simulink model "project_simulink"  (R2024a)
settings: Solver=VariableStepAuto  StartTime=0.0  StopTime=100  RelTol=1e-3
values from neighbouring files (symbols this model uses):
  b = 9.144    [aircraft_6dof.m]
  c = 3.45    [aircraft_6dof.m]
  delta_lef = 0    [aircraft_6dof.m]
  delta_r = 0    [aircraft_6dof.m]
  delta_sb = 0    [aircraft_6dof.m]
  f16_database =     [F16_LookupTables.mat]
  mass = 9300    [aircraft_6dof.m]
  S = 27.88    [aircraft_6dof.m]
  V_c = [153]    [aircraft_6dof.m]
libraries: aerolibconvert2 x5, shared6dof x1, aerolibatmos2 x1, aerolibasang x1
(part 1 of 2)
settings Model: Creator=caner  LastModifiedBy=HUSEYIN
settings OptimizationCC: ReuseModelBlockBuffer=off
settings RTWCC: GPUComputeCapability=3.5

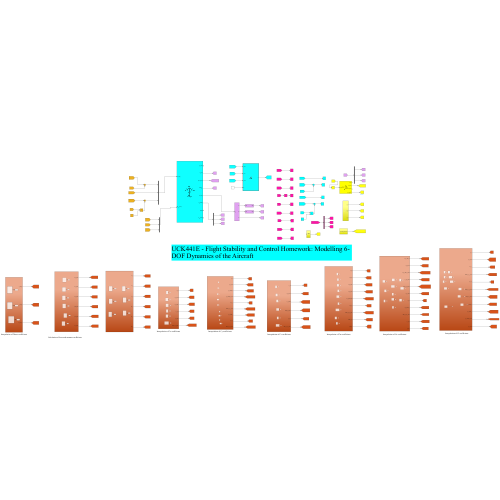
[thumbnail: Simulink's stored preview of the top-level diagram]
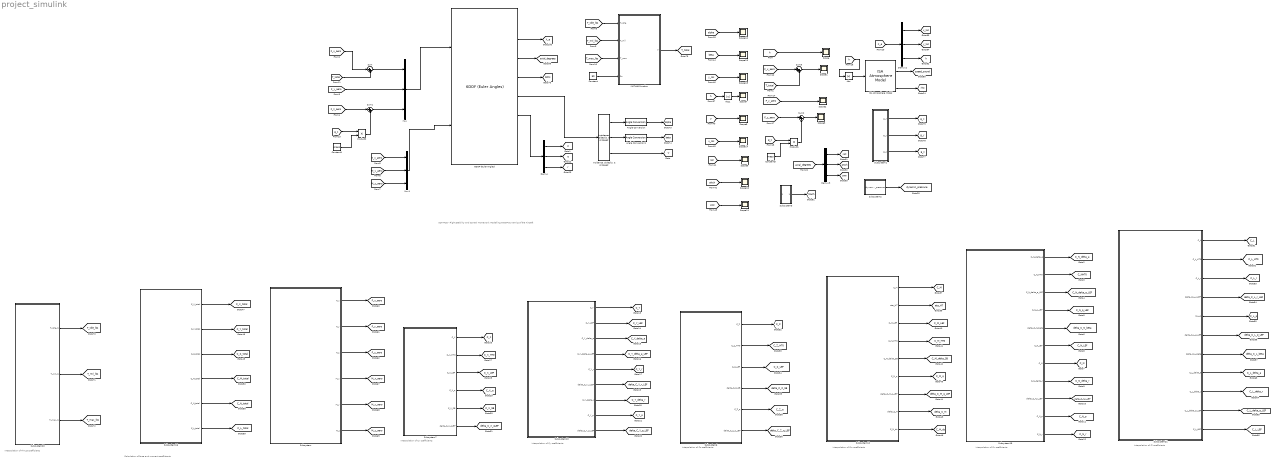
== system project_simulink ==
  note: UCK441E - Flight Stability and Control Homework: Modelling 6-DOF Dynamics of the Aircraft
  note: Interpolation of Cx coefficients
  note: Interpolation of Cy coefficients
  note: Interpolation of Cz coefficients
  note: Interpolation of Cm coefficients
  note: Interpolation of Cn coefficients
  note: Interpolation of Cl coefficients
  note: Interpolation of Thrust coefficients
  note: Calculation of force and moment coefficients
  6DOF (Euler Angles) : shared6dof/6DOF (Euler Angles)  units=Metric (MKS)  mtype=Fixed  rep=Euler Angles  xme_0=[0 0 -3048]  Vm_0=[153 0 0]  eul_0=[0 0 0]  pm_0=[0 0 0]  mass_0=9300  mass_e=0.5  mass_f=2.0  inertia=I  inertia_e=eye(3)  inertia_f=2*eye(3)  k_quat=1.0  vre_flag=on  abi_flag=off  aMode=0  xme_statename=''  Vm_statename=''  eul_statename=''  quat_statename=''  pm_statename=''  mass_statename=''
  Abs : Abs  SaturateOnIntegerOverflow=off
  Abs1 : Abs  SaturateOnIntegerOverflow=off
  Angle Conversion : aerolibconvert2/Angle Conversion  IU=rad  OU=deg
  Angle Conversion1 : aerolibconvert2/Angle Conversion  IU=rad  OU=deg
  Constant : Constant  Value=50
  Constant1 : Constant  Value=mass
  Constant3 : Constant  Value=mass
  Demux : Demux  Outputs=3
  Demux2 : Demux  Outputs=3
  Demux3 : Demux  Outputs=3
  ISA Atmosphere Model : aerolibatmos2/ISA Atmosphere Model  useExtended=off  action=Warning  custom=off  viscosityOut=off  g=9.80665  gamma=1.4  R=287.0531  L=0.0065  h_trop=11000  h_strat=20000  rho0=1.225  P0=101325  T0=288.15  h0=0  S=110.4  Tref=273.15  muref=1.716e-5
  "Incidence, Sideslip, & Airspeed" : aerolibasang/Incidence, Sideslip, & Airspeed
  MATLAB Function : MATLAB Function  TreatAsAtomicUnit=on
  Mux : Mux  Inputs=3
  Mux1 : Mux  Inputs=3
  Product1 : Product
  Product2 : Product
  Scope{,1..3,7..15} (13 alike) : Scope
  Subsystem : Subsystem
  Subsystem1 : Subsystem
  Subsystem10 : Subsystem
  Subsystem12 : Subsystem
  Subsystem15 : Subsystem
  Subsystem16 : Subsystem
  Subsystem2 : Subsystem
  Subsystem20 : Subsystem
  Subsystem21 : Subsystem
  Subsystem3 : Subsystem
  Subsystem6 : Subsystem
  Subsystem7 : Subsystem
  Sum{,1..3} (4 alike) : Sum  Inputs=|++
  tag scope: C_L=global, C_L_HT0=global, C_L_LEF=global, C_L_delta_a=global, C_L_delta_a_LEF=global, C_L_delta_r=global, C_L_p=global, C_L_r=global, C_L_total=global, C_M=global, C_M_HT0=global, C_M_LEF=global, C_M_delta_SB=global, C_M_ds=global, C_M_q=global, C_M_total=global, C_N=global, C_NHT0=global, C_N_LEF=global, C_N_delta_a=global, C_N_delta_a_LEF=global, C_N_delta_r=global, C_N_p=global, C_N_p_LEF=global, C_N_r=global, C_N_total=global, C_X=global, C_X_HT0=global, C_X_LEF=global, C_X_SB=global, C_X_q=global, C_X_total=global, C_Y=global, C_Y_LEF=global, C_Y_delta_a=global, C_Y_delta_a_LEF=global, C_Y_delta_r=global, C_Y_p=global, C_Y_r=global, C_Y_total=global, C_Z=global, C_Z_HT0=global, C_Z_LEF=global, C_Z_q=global, C_Z_total=global, DCM=global, F_x_aero=global, F_y_aero=global, F_z_aero=global, M_x_aero=global, M_y_aero=global, M_z_aero=global, Mach=global, T_idle_lbs=global, T_max_lbs=global, T_mil_lbs=global, T_total=global, V=global, X_e=global, alpha=global, axial_degrees=global, beta=global, delta_C_L_beta=global, delta_C_L_p_LEF=global, delta_C_L_r_LEF=global, delta_C_M=global, delta_C_M_q_LEF=global, delta_C_N_beta=global, delta_C_N_r_LEF=global, delta_C_X_qLEF=global, delta_C_Y_p_LEF=global, delta_C_Y_r_LEF=global, delta_C_Z_SB=global, delta_C_Z_q_LEF=global, dynamic_pressure=global, eta_HT=global, g_x=global, g_y=global, g_z=global, h=global, p=global, pitch=global, q=global, r=global, rho=global, roll=global, speed_sound=global, x_loc=global, y_loc=global, yaw=global
  wires:
  6DOF (Euler Angles)/5 -> "Incidence, Sideslip, & Airspeed"/1
  "Incidence, Sideslip, & Airspeed"/3 -> [V]
  6DOF (Euler Angles)/6 -> Demux/1
  Subsystem15/1(C_N_delta_a) -> [C_N_delta_a]
  Subsystem15/3(C_N_delta_a_LEF) -> [C_N_delta_a_LEF]
  Subsystem15/4(C_N_p_LEF) -> [C_N_p_LEF]
  Subsystem15/5(delta_C_N_beta) -> [delta_C_N_beta]
  Subsystem15/7(C_N) -> [C_N]
  Subsystem15/6(C_N_LEF) -> [C_N_LEF]
  Subsystem15/2(C_N_HT0) -> [C_NHT0]
  Subsystem15/8(C_N_delta_r) -> [C_N_delta_r]
  Subsystem15/9(delta_C_N_r_LEF) -> [delta_C_N_r_LEF]
  Subsystem15/10(C_N_p) -> [C_N_p]
  Subsystem15/11(C_N_r) -> [C_N_r]
  Subsystem10/1(C_Y) -> [C_Y]
  Subsystem10/2(C_Y_LEF) -> [C_Y_LEF]
  Subsystem10/3(C_Y_delta_a) -> [C_Y_delta_a]
  Subsystem10/4(C_Y_delta_a_LEF) -> [C_Y_delta_a_LEF]
  Subsystem10/5(C_Y_r) -> [C_Y_r]
  Subsystem10/6(delta_C_Y_r_LEF) -> [delta_C_Y_r_LEF]
  Subsystem10/7(C_Y_delta_r) -> [C_Y_delta_r]
  Subsystem10/8(C_Y_p) -> [C_Y_p]
  Subsystem10/9(delta_C_Y_p_LEF) -> [delta_C_Y_p_LEF]
  ISA Atmosphere Model/4 -> [rho]
  Subsystem7/1(C_X) -> [C_X]
  Subsystem7/2(C_X_HT0) -> [C_X_HT0]
  Subsystem7/3(C_X_LEF) -> [C_X_LEF]
  Subsystem7/4(C_X_q) -> [C_X_q]
  Subsystem7/5(C_X_SB) -> [C_X_SB]
  Subsystem7/6(delta_C_X_qLEF) -> [delta_C_X_qLEF]
  Subsystem6/1(C_Z) -> [C_Z]
  Subsystem6/2(C_Z_HT0) -> [C_Z_HT0]
  Subsystem6/3(C_Z_LEF) -> [C_Z_LEF]
  Subsystem6/4(delta_C_Z_SB) -> [delta_C_Z_SB]
  Subsystem6/5(C_Z_q) -> [C_Z_q]
  Subsystem6/6(delta_C_Z_q_LEF) -> [delta_C_Z_q_LEF]
  Subsystem12/1(C_M) -> [C_M]
  Subsystem12/2(eta_HT) -> [eta_HT]
  Subsystem12/3(C_M_LEF) -> [C_M_LEF]
  Subsystem12/4(C_M_HT0) -> [C_M_HT0]
  Subsystem12/5(C_M_delta_SB) -> [C_M_delta_SB]
  Subsystem12/6(C_M_q) -> [C_M_q]
  Subsystem12/7(delta_C_M_q_LEF) -> [delta_C_M_q_LEF]
  Subsystem12/8(delta_C_M) -> [delta_C_M]
  Subsystem12/9(C_M_ds) -> [C_M_ds]
  Subsystem21/1(C_L) -> [C_L]
  Subsystem21/2(C_L_HT0) -> [C_L_HT0]
  Subsystem21/3(C_L_r) -> [C_L_r]
  Subsystem21/4(delta_C_L_r_LEF) -> [delta_C_L_r_LEF]
  Subsystem21/5(C_L_p) -> [C_L_p]
  Subsystem21/6(delta_C_L_p_LEF) -> [delta_C_L_p_LEF]
  Subsystem21/7(delta_C_L_beta) -> [delta_C_L_beta]
  Subsystem21/8(C_L_delta_a) -> [C_L_delta_a]
  Subsystem21/9(C_L_delta_r) -> [C_L_delta_r]
  Subsystem21/10(C_L_delta_a_LEF) -> [C_L_delta_a_LEF]
  Subsystem21/11(C_L_LEF) -> [C_L_LEF]
  [F_y_aero] -> Mux/2
  Mux/1 -> 6DOF (Euler Angles)/1
  [M_x_aero] -> Mux1/1
  [M_z_aero] -> Mux1/3
  [M_y_aero] -> Mux1/2
  Mux1/1 -> 6DOF (Euler Angles)/2
  Subsystem20/1(T_idle_N) -> [T_idle_lbs]
  Subsystem20/2(T_mil_N) -> [T_mil_lbs]
  Subsystem20/3(T_max_N) -> [T_max_lbs]
  Subsystem16/1(C_X_total) -> [C_X_total]
  Subsystem16/2(C_Y_total) -> [C_Y_total]
  Subsystem16/3(C_Z_total) -> [C_Z_total]
  Subsystem16/4(C_M_total) -> [C_M_total]
  Subsystem16/5(C_N_total) -> [C_N_total]
  Subsystem16/6(C_L_total) -> [C_L_total]
  Subsystem/1(F_x) -> [F_x_aero]
  Subsystem/2(F_y) -> [F_y_aero]
  Subsystem/3(F_z) -> [F_z_aero]
  Subsystem/4(M_x) -> [M_x_aero]
  Subsystem/5(M_y) -> [M_y_aero]
  Subsystem/6(M_z) -> [M_z_aero]
  "Incidence, Sideslip, & Airspeed"/1 -> Angle Conversion/1
  Angle Conversion/1 -> [alpha]
  "Incidence, Sideslip, & Airspeed"/2 -> Angle Conversion1/1
  Angle Conversion1/1 -> [beta]
  Demux/1 -> [p]
  Demux/2 -> [q]
  Demux/3 -> [r]
  [T_idle_lbs] -> MATLAB Function/1(T_idle)
  [T_mil_lbs] -> MATLAB Function/2(T_mil)
  [T_max_lbs] -> MATLAB Function/3(T_max)
  Constant/1 -> MATLAB Function/4(Pc)
  MATLAB Function/1(T) -> [T_total]
  [F_x_aero] -> Sum/1
  [T_total] -> Sum/2
  Sum/1 -> Mux/1
  6DOF (Euler Angles)/4 -> [DCM]
  [F_z_aero] -> Sum1/1
  [g_z] -> Product2/1
  Constant1/1 -> Product2/2
  Sum1/1 -> Mux/3
  Product2/1 -> Sum1/2
  ISA Atmosphere Model/2 -> [speed_sound]
  Demux2/3 -> [h]
  Demux2/1 -> [x_loc]
  Demux2/2 -> [y_loc]
  Subsystem1/1(g_x) -> [g_x]
  Subsystem1/2(g_y) -> [g_y]
  Subsystem1/3(g_z) -> [g_z]
  Subsystem2/1(dynamic_pressure) -> [dynamic_pressure]
  Subsystem3/1(Mach) -> [Mach]
  [T_total] -> Sum3/2
  [F_x_aero] -> Sum3/1
  Product1/1 -> Sum2/2
  Sum2/1 -> Scope3/1
  Constant3/1 -> Product1/2
  [F_z_aero] -> Sum2/1
  [g_z] -> Product1/1
  Sum3/1 -> Scope1/1
  [F_y_aero] -> Scope2/1
  [h] -> Abs/1
  Abs/1 -> ISA Atmosphere Model/1
  [h] -> Scope/1
  6DOF (Euler Angles)/2 -> [X_e]
  [X_e] -> Demux2/1
  6DOF (Euler Angles)/3 -> [axial_degrees]
  [axial_degrees] -> Demux3/1
  Demux3/1 -> [roll]
  Demux3/2 -> [pitch]
  Demux3/3 -> [yaw]
  [V] -> Scope8/1
  Abs1/1 -> Scope7/1
  [h] -> Abs1/1
  [roll] -> Scope9/1
  [pitch] -> Scope10/1
  [yaw] -> Scope11/1
  [alpha] -> Scope12/1
  [beta] -> Scope13/1
  [x_loc] -> Scope14/1
  [y_loc] -> Scope15/1

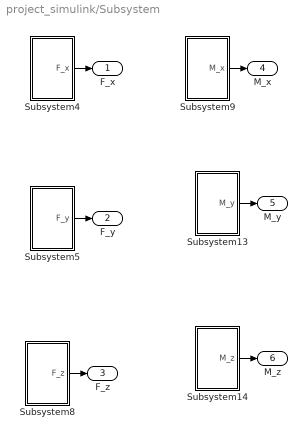
== system project_simulink/Subsystem ==
  Subsystem13 : Subsystem
  Subsystem14 : Subsystem
  Subsystem4 : Subsystem
  Subsystem5 : Subsystem
  Subsystem8 : Subsystem
  Subsystem9 : Subsystem
  F_x : Outport
  F_y : Outport  Port=2
  F_z : Outport  Port=3
  M_x : Outport  Port=4
  M_y : Outport  Port=5
  M_z : Outport  Port=6
  wires:
  Subsystem14/1(M_z) -> M_z/1
  Subsystem4/1(F_x) -> F_x/1
  Subsystem8/1(F_z) -> F_z/1
  Subsystem13/1(M_y) -> M_y/1
  Subsystem5/1(F_y) -> F_y/1
  Subsystem9/1(M_x) -> M_x/1

== system project_simulink/Subsystem1 ==
  Demux1 : Demux  Outputs=3
  Product1 : Product  Multiplication=Matrix(*)
  gravitational acceleration : Constant  Value=[0,0,9.81]
  g_x : Outport
  g_y : Outport  Port=2
  g_z : Outport  Port=3
  wires:
  gravitational acceleration/1 -> Product1/2
  Demux1/2 -> g_y/1  "g_y"
  Product1/1 -> Demux1/1
  Demux1/3 -> g_z/1  "g_z"
  [DCM] -> Product1/1
  Demux1/1 -> g_x/1  "g_x"

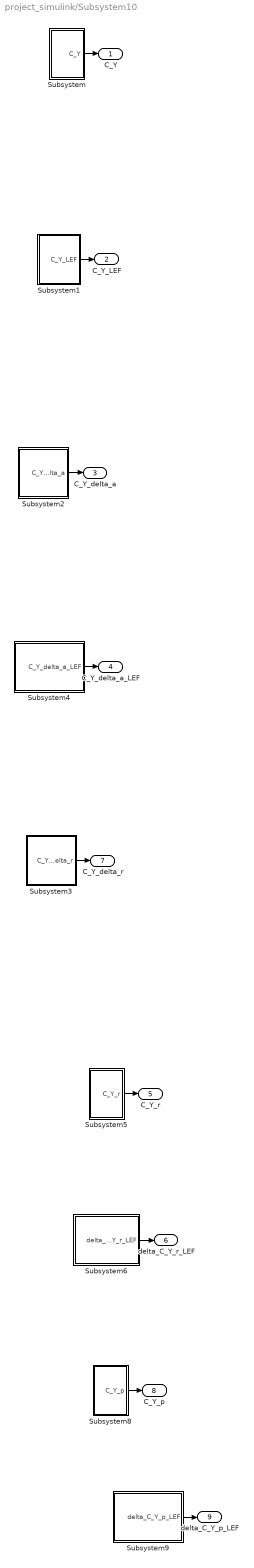
== system project_simulink/Subsystem10 ==
  Subsystem : Subsystem
  Subsystem1 : Subsystem
  Subsystem2 : Subsystem
  Subsystem3 : Subsystem
  Subsystem4 : Subsystem
  Subsystem5 : Subsystem
  Subsystem6 : Subsystem
  Subsystem8 : Subsystem
  Subsystem9 : Subsystem
  C_Y : Outport
  C_Y_LEF : Outport  Port=2
  C_Y_delta_a : Outport  Port=3
  C_Y_delta_a_LEF : Outport  Port=4
  C_Y_r : Outport  Port=5
  delta_C_Y_r_LEF : Outport  Port=6
  C_Y_delta_r : Outport  Port=7
  C_Y_p : Outport  Port=8
  delta_C_Y_p_LEF : Outport  Port=9
  wires:
  Subsystem2/1(C_Y_delta_a) -> C_Y_delta_a/1
  Subsystem/1(C_Y) -> C_Y/1
  Subsystem1/1(C_Y_LEF) -> C_Y_LEF/1
  Subsystem6/1(delta_C_Y_r_LEF) -> delta_C_Y_r_LEF/1
  Subsystem4/1(C_Y_delta_a_LEF) -> C_Y_delta_a_LEF/1
  Subsystem9/1(delta_C_Y_p_LEF) -> delta_C_Y_p_LEF/1
  Subsystem5/1(C_Y_r) -> C_Y_r/1
  Subsystem3/1(C_Y_delta_r) -> C_Y_delta_r/1
  Subsystem8/1(C_Y_p) -> C_Y_p/1

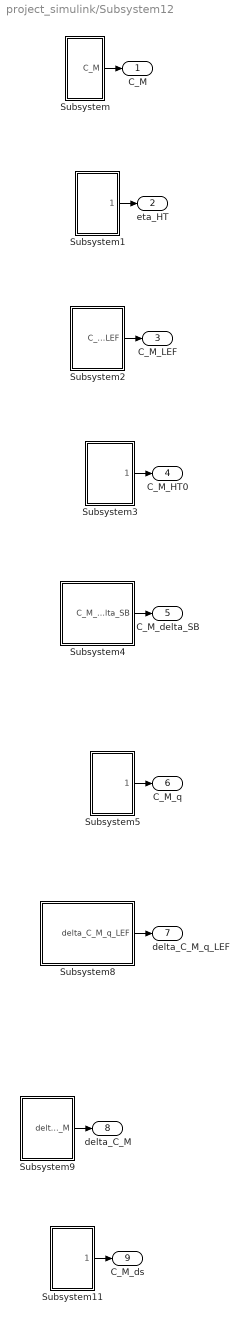
== system project_simulink/Subsystem12 ==
  Subsystem : Subsystem
  Subsystem1 : Subsystem
  Subsystem11 : Subsystem
  Subsystem2 : Subsystem
  Subsystem3 : Subsystem
  Subsystem4 : Subsystem
  Subsystem5 : Subsystem
  Subsystem8 : Subsystem
  Subsystem9 : Subsystem
  C_M : Outport
  eta_HT : Outport  Port=2
  C_M_LEF : Outport  Port=3
  C_M_HT0 : Outport  Port=4
  C_M_delta_SB : Outport  Port=5
  C_M_q : Outport  Port=6
  delta_C_M_q_LEF : Outport  Port=7
  delta_C_M : Outport  Port=8
  C_M_ds : Outport  Port=9
  wires:
  Subsystem4/1(C_M_delta_SB) -> C_M_delta_SB/1
  Subsystem5/1(C_M_q) -> C_M_q/1
  Subsystem8/1(delta_C_M_q_LEF) -> delta_C_M_q_LEF/1
  Subsystem1/1(eta_HT) -> eta_HT/1
  Subsystem11/1(C_M_ds) -> C_M_ds/1
  Subsystem/1(C_M) -> C_M/1
  Subsystem3/1(C_M_HT0) -> C_M_HT0/1
  Subsystem2/1(C_M_LEF) -> C_M_LEF/1
  Subsystem9/1(delta_C_M) -> delta_C_M/1

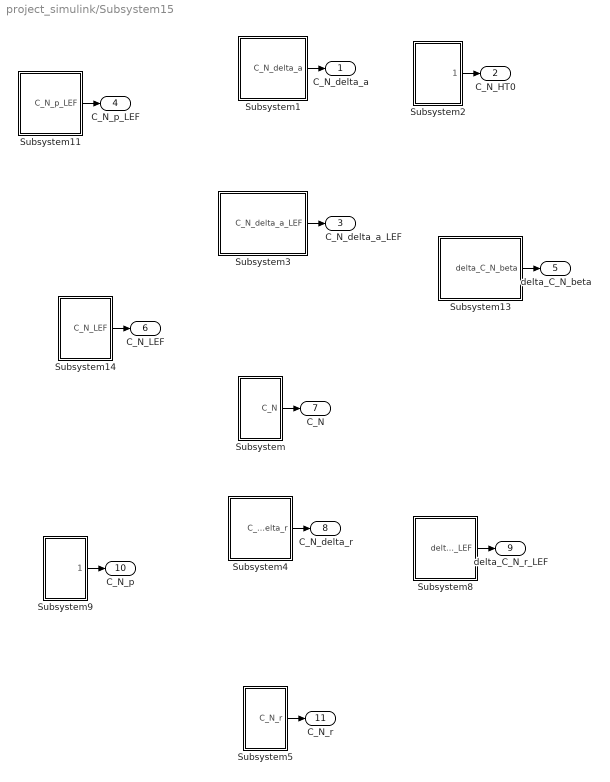
== system project_simulink/Subsystem15 ==
  Subsystem : Subsystem
  Subsystem1 : Subsystem
  Subsystem11 : Subsystem
  Subsystem13 : Subsystem
  Subsystem14 : Subsystem
  Subsystem2 : Subsystem
  Subsystem3 : Subsystem
  Subsystem4 : Subsystem
  Subsystem5 : Subsystem
  Subsystem8 : Subsystem
  Subsystem9 : Subsystem
  C_N_delta_a : Outport
  C_N_HT0 : Outport  Port=2
  C_N_delta_a_LEF : Outport  Port=3
  C_N_p_LEF : Outport  Port=4
  delta_C_N_beta : Outport  Port=5
  C_N_LEF : Outport  Port=6
  C_N : Outport  Port=7
  C_N_delta_r : Outport  Port=8
  delta_C_N_r_LEF : Outport  Port=9
  C_N_p : Outport  Port=10
  C_N_r : Outport  Port=11
  wires:
  Subsystem2/1(C_N_HT0) -> C_N_HT0/1
  Subsystem5/1(C_N_r) -> C_N_r/1
  Subsystem14/1(C_N_LEF) -> C_N_LEF/1
  Subsystem4/1(C_N_delta_r) -> C_N_delta_r/1
  Subsystem/1(C_N) -> C_N/1
  Subsystem3/1(C_N_delta_a_LEF) -> C_N_delta_a_LEF/1
  Subsystem11/1(C_N_p_LEF) -> C_N_p_LEF/1
  Subsystem9/1(C_N_p) -> C_N_p/1
  Subsystem13/1(delta_C_N_beta) -> delta_C_N_beta/1
  Subsystem1/1(C_N_delta_a) -> C_N_delta_a/1
  Subsystem8/1(delta_C_N_r_LEF) -> delta_C_N_r_LEF/1

== system project_simulink/Subsystem16 ==
  Subsystem : Subsystem
  Subsystem1 : Subsystem
  Subsystem11 : Subsystem
  Subsystem18 : Subsystem
  Subsystem2 : Subsystem
  Subsystem3 : Subsystem
  C_X_total : Outport
  C_Y_total : Outport  Port=2
  C_Z_total : Outport  Port=3
  C_M_total : Outport  Port=4
  C_N_total : Outport  Port=5
  C_L_total : Outport  Port=6
  wires:
  Subsystem18/1(C_L_total) -> C_L_total/1
  Subsystem/1(C_Y_total) -> C_Y_total/1
  Subsystem1/1(C_X_total) -> C_X_total/1
  Subsystem11/1(C_N_total) -> C_N_total/1
  Subsystem3/1(C_M_total) -> C_M_total/1
  Subsystem2/1(C_Z_total) -> C_Z_total/1

== system project_simulink/Subsystem2 ==
  Multiply : Gain  Gain=1/2
  Product : Product
  Square : Math  Operator=square
  dynamic_pressure : Outport
  wires:
  [rho] -> Product/2
  Multiply/1 -> Product/1
  Square/1 -> Multiply/1
  Product/1 -> dynamic_pressure/1  "dynamic_pressure"
  [V] -> Square/1

== system project_simulink/Subsystem20 ==
  Subsystem16 : Subsystem
  Subsystem17 : Subsystem
  Subsystem19 : Subsystem
  T_idle_N : Outport
  T_mil_N : Outport  Port=2
  T_max_N : Outport  Port=3
  wires:
  Subsystem17/1(T_mil_N) -> T_mil_N/1
  Subsystem19/1(T_max_N) -> T_max_N/1
  Subsystem16/1(T_idle_N) -> T_idle_N/1

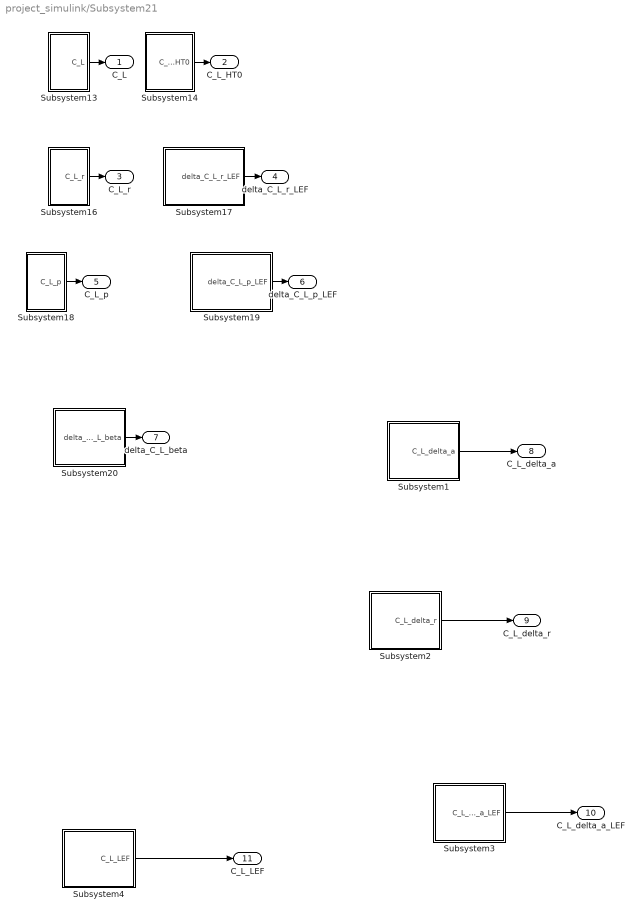
== system project_simulink/Subsystem21 ==
  Subsystem1 : Subsystem
  Subsystem13 : Subsystem
  Subsystem14 : Subsystem
  Subsystem16 : Subsystem
  Subsystem17 : Subsystem
  Subsystem18 : Subsystem
  Subsystem19 : Subsystem
  Subsystem2 : Subsystem
  Subsystem20 : Subsystem
  Subsystem3 : Subsystem
  Subsystem4 : Subsystem
  C_L : Outport
  C_L_HT0 : Outport  Port=2
  C_L_r : Outport  Port=3
  delta_C_L_r_LEF : Outport  Port=4
  C_L_p : Outport  Port=5
  delta_C_L_p_LEF : Outport  Port=6
  delta_C_L_beta : Outport  Port=7
  C_L_delta_a : Outport  Port=8
  C_L_delta_r : Outport  Port=9
  C_L_delta_a_LEF : Outport  Port=10
  C_L_LEF : Outport  Port=11
  wires:
  Subsystem20/1(delta_C_L_beta) -> delta_C_L_beta/1
  Subsystem18/1(C_L_p) -> C_L_p/1
  Subsystem14/1(C_L_HT0) -> C_L_HT0/1
  Subsystem19/1(delta_C_L_p_LEF) -> delta_C_L_p_LEF/1
  Subsystem16/1(C_L_r) -> C_L_r/1
  Subsystem17/1(delta_C_L_r_LEF) -> delta_C_L_r_LEF/1
  Subsystem13/1(C_L) -> C_L/1
  Subsystem1/1(C_L_delta_a) -> C_L_delta_a/1
  Subsystem2/1(C_L_delta_r) -> C_L_delta_r/1
  Subsystem3/1(C_L_delta_a_LEF) -> C_L_delta_a_LEF/1
  Subsystem4/1(C_L_LEF) -> C_L_LEF/1

== system project_simulink/Subsystem3 ==
  In1 : Inport
  Divide : Product  Inputs=*/
  Mach : Outport
  wires:
  Divide/1 -> Mach/1  "Mach"
  [speed_sound] -> Divide/2
  [V] -> Divide/1

== system project_simulink/Subsystem6 ==
  Subsystem : Subsystem
  Subsystem1 : Subsystem
  Subsystem2 : Subsystem
  Subsystem3 : Subsystem
  Subsystem4 : Subsystem
  Subsystem5 : Subsystem
  C_Z : Outport
  C_Z_HT0 : Outport  Port=2
  C_Z_LEF : Outport  Port=3
  delta_C_Z_SB : Outport  Port=4
  C_Z_q : Outport  Port=5
  delta_C_Z_q_LEF : Outport  Port=6
  wires:
  Subsystem5/1(delta_C_Z_q_LEF) -> delta_C_Z_q_LEF/1
  Subsystem1/1(C_Z_HT0) -> C_Z_HT0/1
  Subsystem3/1(delta_C_Z_SB) -> delta_C_Z_SB/1
  Subsystem4/1(C_Z_q) -> C_Z_q/1
  Subsystem/1(C_Z) -> C_Z/1
  Subsystem2/1(C_Z_LEF) -> C_Z_LEF/1

== system project_simulink/Subsystem7 ==
  Subsystem : Subsystem
  Subsystem1 : Subsystem
  Subsystem2 : Subsystem
  Subsystem3 : Subsystem
  Subsystem4 : Subsystem
  Subsystem5 : Subsystem
  C_X : Outport
  C_X_HT0 : Outport  Port=2
  C_X_LEF : Outport  Port=3
  C_X_q : Outport  Port=4
  C_X_SB : Outport  Port=5
  delta_C_X_qLEF : Outport  Port=6
  wires:
  Subsystem1/1(C_X_HT0) -> C_X_HT0/1
  Subsystem/1(C_X) -> C_X/1
  Subsystem2/1(C_X_LEF) -> C_X_LEF/1
  Subsystem3/1(C_X_q) -> C_X_q/1
  Subsystem4/1(C_X_SB) -> C_X_SB/1
  Subsystem5/1(delta_C_X_qLEF) -> delta_C_X_qLEF/1

== system project_simulink/Subsystem/Subsystem13 ==
  Constant : Constant  Value=c
  Constant1 : Constant  Value=S
  Product1 : Product  Inputs=4
  M_y : Outport
  wires:
  Constant1/1 -> Product1/2
  [dynamic_pressure] -> Product1/1
  [C_N_total] -> Product1/3
  Product1/1 -> M_y/1  "M_y"
  Constant/1 -> Product1/4

== system project_simulink/Subsystem/Subsystem14 ==
  Constant : Constant  Value=b
  Constant1 : Constant  Value=S
  Product1 : Product  Inputs=4
  M_z : Outport
  wires:
  Constant1/1 -> Product1/2
  [dynamic_pressure] -> Product1/1
  [C_L_total] -> Product1/3
  Product1/1 -> M_z/1  "M_z"
  Constant/1 -> Product1/4

== system project_simulink/Subsystem/Subsystem4 ==
  Constant1 : Constant  Value=S
  Product1 : Product  Inputs=3
  F_x : Outport
  wires:
  Constant1/1 -> Product1/2
  [dynamic_pressure] -> Product1/1
  [C_X_total] -> Product1/3
  Product1/1 -> F_x/1  "F_x"

== system project_simulink/Subsystem/Subsystem5 ==
  Constant1 : Constant  Value=S
  Product1 : Product  Inputs=3
  F_y : Outport
  wires:
  Constant1/1 -> Product1/2
  [dynamic_pressure] -> Product1/1
  [C_Y_total] -> Product1/3
  Product1/1 -> F_y/1  "F_y"

== system project_simulink/Subsystem/Subsystem8 ==
  Constant1 : Constant  Value=S
  Product1 : Product  Inputs=3
  F_z : Outport
  wires:
  Constant1/1 -> Product1/2
  [dynamic_pressure] -> Product1/1
  [C_Z_total] -> Product1/3
  Product1/1 -> F_z/1  "F_z"

== system project_simulink/Subsystem/Subsystem9 ==
  Constant : Constant  Value=b
  Constant1 : Constant  Value=S
  Product1 : Product  Inputs=4
  M_x : Outport
  wires:
  Constant1/1 -> Product1/2
  [dynamic_pressure] -> Product1/1
  [C_M_total] -> Product1/3
  Product1/1 -> M_x/1  "M_x"
  Constant/1 -> Product1/4

== system project_simulink/Subsystem10/Subsystem ==
  Interpolation Using Prelookup : Interpolation_n-D  Table=f16_database.f16_AerodynamicData.data.CY.CY  InternalRulePriority=Speed
  Prelookup : PreLookup  BreakpointsData=f16_database.f16_AerodynamicData.BP.CY.CY.alpha  ExtrapMethod=Linear
  Prelookup1 : PreLookup  BreakpointsData=f16_database.f16_AerodynamicData.BP.CY.CY.beta  ExtrapMethod=Linear
  C_Y : Outport
  wires:
  Prelookup/2 -> Interpolation Using Prelookup/2
  [beta] -> Prelookup1/1
  Prelookup1/2 -> Interpolation Using Prelookup/4
  [alpha] -> Prelookup/1
  Prelookup1/1 -> Interpolation Using Prelookup/3
  Prelookup/1 -> Interpolation Using Prelookup/1
  Interpolation Using Prelookup/1 -> C_Y/1  "C_Y"

== system project_simulink/Subsystem10/Subsystem1 ==
  Interpolation Using Prelookup1 : Interpolation_n-D  Table=f16_database.f16_AerodynamicData.data.CY.CYlef  InternalRulePriority=Speed
  Prelookup2 : PreLookup  BreakpointsData=f16_database.f16_AerodynamicData.BP.CY.CYlef.alpha  ExtrapMethod=Linear
  Prelookup3 : PreLookup  BreakpointsData=f16_database.f16_AerodynamicData.BP.CY.CYlef.beta  ExtrapMethod=Linear
  C_Y_LEF : Outport
  wires:
  [beta] -> Prelookup3/1
  [alpha] -> Prelookup2/1
  Prelookup3/2 -> Interpolation Using Prelookup1/4
  Prelookup2/2 -> Interpolation Using Prelookup1/2
  Prelookup2/1 -> Interpolation Using Prelookup1/1
  Prelookup3/1 -> Interpolation Using Prelookup1/3
  Interpolation Using Prelookup1/1 -> C_Y_LEF/1  "C_Y_LEF"

== system project_simulink/Subsystem10/Subsystem2 ==
  Interpolation Using Prelookup2 : Interpolation_n-D  Table=f16_database.f16_AerodynamicData.data.CY.CYda20  InternalRulePriority=Speed
  Prelookup4 : PreLookup  BreakpointsData=f16_database.f16_AerodynamicData.BP.CY.CYda20.alpha  ExtrapMethod=Linear
  Prelookup5 : PreLookup  BreakpointsData=f16_database.f16_AerodynamicData.BP.CY.CYda20.beta  ExtrapMethod=Linear
  C_Y_delta_a : Outport
  wires:
  Interpolation Using Prelookup2/1 -> C_Y_delta_a/1  "C_Y_delta_a"
  Prelookup4/2 -> Interpolation Using Prelookup2/2
  [alpha] -> Prelookup4/1
  [beta] -> Prelookup5/1
  Prelookup4/1 -> Interpolation Using Prelookup2/1
  Prelookup5/1 -> Interpolation Using Prelookup2/3
  Prelookup5/2 -> Interpolation Using Prelookup2/4

== system project_simulink/Subsystem10/Subsystem3 ==
  Interpolation Using Prelookup4 : Interpolation_n-D  Table=f16_database.f16_AerodynamicData.data.CY.CYdr30  InternalRulePriority=Speed
  Prelookup8 : PreLookup  BreakpointsData=f16_database.f16_AerodynamicData.BP.CY.CYdr30.alpha  ExtrapMethod=Linear
  Prelookup9 : PreLookup  BreakpointsData=f16_database.f16_AerodynamicData.BP.CY.CYdr30.beta  ExtrapMethod=Linear
  C_Y_delta_r : Outport
  wires:
  Prelookup8/1 -> Interpolation Using Prelookup4/1
  Interpolation Using Prelookup4/1 -> C_Y_delta_r/1  "C_Y_delta_r"
  Prelookup9/2 -> Interpolation Using Prelookup4/4
  [beta] -> Prelookup9/1
  Prelookup8/2 -> Interpolation Using Prelookup4/2
  Prelookup9/1 -> Interpolation Using Prelookup4/3
  [alpha] -> Prelookup8/1

== system project_simulink/Subsystem10/Subsystem4 ==
  Subsystem3 : Subsystem
  C_Y_delta_a_LEF : Outport
  wires:
  Subsystem3/1(C_Y_delta_a_LEF) -> C_Y_delta_a_LEF/1

== system project_simulink/Subsystem10/Subsystem5 ==
  Interpolation Using Prelookup5 : Interpolation_n-D  NumberOfTableDimensions=1  Table=f16_database.f16_AerodynamicData.data.CY.CYr  InternalRulePriority=Speed
      settings: InputPortMap=u0,u1
  Prelookup10 : PreLookup  BreakpointsData=f16_database.f16_AerodynamicData.BP.CY.CYr.alpha  ExtrapMethod=Linear
  C_Y_r : Outport
  wires:
  [alpha] -> Prelookup10/1
  Prelookup10/2 -> Interpolation Using Prelookup5/2
  Prelookup10/1 -> Interpolation Using Prelookup5/1
  Interpolation Using Prelookup5/1 -> C_Y_r/1  "C_Y_r"

== system project_simulink/Subsystem10/Subsystem6 ==
  Interpolation Using Prelookup6 : Interpolation_n-D  NumberOfTableDimensions=1  Table=f16_database.f16_AerodynamicData.data.CY.deltaCYrlef  InternalRulePriority=Speed
      settings: InputPortMap=u0,u1
  Prelookup11 : PreLookup  BreakpointsData=f16_database.f16_AerodynamicData.BP.CY.deltaCYrlef.alpha  ExtrapMethod=Linear
  delta_C_Y_r_LEF : Outport
  wires:
  [alpha] -> Prelookup11/1
  Interpolation Using Prelookup6/1 -> delta_C_Y_r_LEF/1  "delta_C_Y_r_LEF"
  Prelookup11/1 -> Interpolation Using Prelookup6/1
  Prelookup11/2 -> Interpolation Using Prelookup6/2

== system project_simulink/Subsystem10/Subsystem8 ==
  Interpolation Using Prelookup7 : Interpolation_n-D  NumberOfTableDimensions=1  Table=f16_database.f16_AerodynamicData.data.CY.CYp  InternalRulePriority=Speed
      settings: InputPortMap=u0,u1
  Prelookup12 : PreLookup  BreakpointsData=f16_database.f16_AerodynamicData.BP.CY.CYp.alpha  ExtrapMethod=Linear
  C_Y_p : Outport
  wires:
  Prelookup12/2 -> Interpolation Using Prelookup7/2
  [alpha] -> Prelookup12/1
  Prelookup12/1 -> Interpolation Using Prelookup7/1
  Interpolation Using Prelookup7/1 -> C_Y_p/1  "C_Y_p"

== system project_simulink/Subsystem10/Subsystem9 ==
  Interpolation Using Prelookup8 : Interpolation_n-D  NumberOfTableDimensions=1  Table=f16_database.f16_AerodynamicData.data.CY.deltaCYplef  InternalRulePriority=Speed
      settings: InputPortMap=u0,u1
  Prelookup13 : PreLookup  BreakpointsData=f16_database.f16_AerodynamicData.BP.CY.deltaCYplef.alpha  ExtrapMethod=Linear
  delta_C_Y_p_LEF : Outport
  wires:
  Prelookup13/1 -> Interpolation Using Prelookup8/1
  Prelookup13/2 -> Interpolation Using Prelookup8/2
  [alpha] -> Prelookup13/1
  Interpolation Using Prelookup8/1 -> delta_C_Y_p_LEF/1  "delta_C_Y_p_LEF"

== system project_simulink/Subsystem12/Subsystem ==
  Interpolation Using Prelookup7 : Interpolation_n-D  NumberOfTableDimensions=3  Table=f16_database.f16_AerodynamicData.data.Cm.Cm  InternalRulePriority=Speed
      settings: InputPortMap=u0,u1,u2,u3,u4,u5
  Prelookup12 : PreLookup  BreakpointsData=f16_database.f16_AerodynamicData.BP.Cm.Cm.dHT  ExtrapMethod=Linear
  Prelookup13 : PreLookup  BreakpointsData=f16_database.f16_AerodynamicData.BP.Cm.Cm.alpha  ExtrapMethod=Linear
  Prelookup14 : PreLookup  BreakpointsData=f16_database.f16_AerodynamicData.BP.Cm.Cm.beta  ExtrapMethod=Linear
  C_M : Outport
  wires:
  Prelookup14/2 -> Interpolation Using Prelookup7/4
  [delta_e] -> Prelookup12/1
  Prelookup13/2 -> Interpolation Using Prelookup7/2
  [alpha] -> Prelookup13/1
  Prelookup13/1 -> Interpolation Using Prelookup7/1
  Prelookup12/1 -> Interpolation Using Prelookup7/5
  Prelookup12/2 -> Interpolation Using Prelookup7/6
  [beta] -> Prelookup14/1
  Prelookup14/1 -> Interpolation Using Prelookup7/3
  Interpolation Using Prelookup7/1 -> C_M/1  "C_M"

== system project_simulink/Subsystem12/Subsystem1 ==
  Interpolation Using Prelookup1 : Interpolation_n-D  NumberOfTableDimensions=1  Table=f16_database.f16_AerodynamicData.data.Cm.n_dHT  InternalRulePriority=Speed
      settings: InputPortMap=u0,u1
  Prelookup1 : PreLookup  BreakpointsData=f16_database.f16_AerodynamicData.BP.Cm.n_dHT.dHT  ExtrapMethod=Linear
  eta_HT : Outport
  wires:
  [delta_e] -> Prelookup1/1
  Interpolation Using Prelookup1/1 -> eta_HT/1  "eta_HT"
  Prelookup1/1 -> Interpolation Using Prelookup1/1
  Prelookup1/2 -> Interpolation Using Prelookup1/2

== system project_simulink/Subsystem12/Subsystem11 ==
  Interpolation Using Prelookup9 : Interpolation_n-D  Table=f16_database.f16_AerodynamicData.data.Cm.deltaCmds  InternalRulePriority=Speed
  Prelookup10 : PreLookup  BreakpointsData=f16_database.f16_AerodynamicData.BP.Cm.deltaCmds.dHT  ExtrapMethod=Linear
  Prelookup9 : PreLookup  BreakpointsData=f16_database.f16_AerodynamicData.BP.Cm.deltaCmds.alpha  ExtrapMethod=Linear
  C_M_ds : Outport
  wires:
  [delta_e] -> Prelookup10/1
  Prelookup10/1 -> Interpolation Using Prelookup9/3
  [alpha] -> Prelookup9/1
  Prelookup9/2 -> Interpolation Using Prelookup9/2
  Prelookup10/2 -> Interpolation Using Prelookup9/4
  Prelookup9/1 -> Interpolation Using Prelookup9/1
  Interpolation Using Prelookup9/1 -> C_M_ds/1  "C_M_ds"

== system project_simulink/Subsystem12/Subsystem2 ==
  Interpolation Using Prelookup8 : Interpolation_n-D  Table=f16_database.f16_AerodynamicData.data.Cm.Cmlef  InternalRulePriority=Speed
  Prelookup15 : PreLookup  BreakpointsData=f16_database.f16_AerodynamicData.BP.Cm.Cmlef.alpha  ExtrapMethod=Linear
  Prelookup16 : PreLookup  BreakpointsData=f16_database.f16_AerodynamicData.BP.Cm.Cmlef.beta  ExtrapMethod=Linear
  C_M_LEF : Outport
  wires:
  Prelookup16/2 -> Interpolation Using Prelookup8/4
  [beta] -> Prelookup16/1
  Prelookup15/2 -> Interpolation Using Prelookup8/2
  [alpha] -> Prelookup15/1
  Prelookup15/1 -> Interpolation Using Prelookup8/1
  Interpolation Using Prelookup8/1 -> C_M_LEF/1  "C_M_LEF"
  Prelookup16/1 -> Interpolation Using Prelookup8/3

== system project_simulink/Subsystem12/Subsystem3 ==
  Constant2 : Constant  Value=0
  Interpolation Using Prelookup2 : Interpolation_n-D  NumberOfTableDimensions=3  Table=f16_database.f16_AerodynamicData.data.Cm.Cm  InternalRulePriority=Speed
      settings: InputPortMap=u0,u1,u2,u3,u4,u5
  Prelookup2 : PreLookup  BreakpointsData=f16_database.f16_AerodynamicData.BP.Cm.Cm.dHT  ExtrapMethod=Linear
  Prelookup3 : PreLookup  BreakpointsData=f16_database.f16_AerodynamicData.BP.Cm.Cm.alpha  ExtrapMethod=Linear
  Prelookup4 : PreLookup  BreakpointsData=f16_database.f16_AerodynamicData.BP.Cm.Cm.beta  ExtrapMethod=Linear
  C_M_HT0 : Outport
  wires:
  Prelookup4/1 -> Interpolation Using Prelookup2/3
  Prelookup2/2 -> Interpolation Using Prelookup2/6
  Prelookup3/1 -> Interpolation Using Prelookup2/1
  Prelookup2/1 -> Interpolation Using Prelookup2/5
  Prelookup4/2 -> Interpolation Using Prelookup2/4
  [beta] -> Prelookup4/1
  Constant2/1 -> Prelookup2/1
  Prelookup3/2 -> Interpolation Using Prelookup2/2
  [alpha] -> Prelookup3/1
  Interpolation Using Prelookup2/1 -> C_M_HT0/1  "C_M_HT0"

== system project_simulink/Subsystem12/Subsystem4 ==
  Interpolation Using Prelookup3 : Interpolation_n-D  NumberOfTableDimensions=1  Table=f16_database.f16_AerodynamicData.data.Cm.deltaCmSB  InternalRulePriority=Speed
      settings: InputPortMap=u0,u1
  Prelookup5 : PreLookup  BreakpointsData=f16_database.f16_AerodynamicData.BP.Cm.deltaCmSB.alpha  ExtrapMethod=Linear
  C_M_delta_SB : Outport
  wires:
  Prelookup5/1 -> Interpolation Using Prelookup3/1
  Prelookup5/2 -> Interpolation Using Prelookup3/2
  [alpha] -> Prelookup5/1
  Interpolation Using Prelookup3/1 -> C_M_delta_SB/1  "C_M_delta_SB"

== system project_simulink/Subsystem12/Subsystem5 ==
  Interpolation Using Prelookup4 : Interpolation_n-D  NumberOfTableDimensions=1  Table=f16_database.f16_AerodynamicData.data.Cm.Cmq  InternalRulePriority=Speed
      settings: InputPortMap=u0,u1
  Prelookup6 : PreLookup  BreakpointsData=f16_database.f16_AerodynamicData.BP.Cm.Cmq.alpha  ExtrapMethod=Linear
  C_M_q : Outport
  wires:
  Interpolation Using Prelookup4/1 -> C_M_q/1  "C_M_q"
  Prelookup6/2 -> Interpolation Using Prelookup4/2
  [alpha] -> Prelookup6/1
  Prelookup6/1 -> Interpolation Using Prelookup4/1

== system project_simulink/Subsystem12/Subsystem8 ==
  Interpolation Using Prelookup5 : Interpolation_n-D  NumberOfTableDimensions=1  Table=f16_database.f16_AerodynamicData.data.Cm.deltaCmqlef  InternalRulePriority=Speed
      settings: InputPortMap=u0,u1
  Prelookup7 : PreLookup  BreakpointsData=f16_database.f16_AerodynamicData.BP.Cm.deltaCmqlef.alpha  ExtrapMethod=Linear
  delta_C_M_q_LEF : Outport
  wires:
  Interpolation Using Prelookup5/1 -> delta_C_M_q_LEF/1  "delta_C_M_q_LEF"
  Prelookup7/2 -> Interpolation Using Prelookup5/2
  Prelookup7/1 -> Interpolation Using Prelookup5/1
  [alpha] -> Prelookup7/1

== system project_simulink/Subsystem12/Subsystem9 ==
  Interpolation Using Prelookup6 : Interpolation_n-D  NumberOfTableDimensions=1  Table=f16_database.f16_AerodynamicData.data.Cm.deltaCm  InternalRulePriority=Speed
      settings: InputPortMap=u0,u1
  Prelookup8 : PreLookup  BreakpointsData=f16_database.f16_AerodynamicData.BP.Cm.deltaCm.alpha  ExtrapMethod=Linear
  delta_C_M : Outport
  wires:
  Prelookup8/1 -> Interpolation Using Prelookup6/1
  Interpolation Using Prelookup6/1 -> delta_C_M/1  "delta_C_M"
  [alpha] -> Prelookup8/1
  Prelookup8/2 -> Interpolation Using Prelookup6/2

== system project_simulink/Subsystem15/Subsystem ==
  Interpolation Using Prelookup1 : Interpolation_n-D  NumberOfTableDimensions=3  Table=f16_database.f16_AerodynamicData.data.Cn.Cn  InternalRulePriority=Speed
      settings: InputPortMap=u0,u1,u2,u3,u4,u5
  Prelookup3 : PreLookup  BreakpointsData=f16_database.f16_AerodynamicData.BP.Cn.Cn.alpha  ExtrapMethod=Linear
  Prelookup4 : PreLookup  BreakpointsData=f16_database.f16_AerodynamicData.BP.Cn.Cn.beta  ExtrapMethod=Linear
  Prelookup5 : PreLookup  BreakpointsData=f16_database.f16_AerodynamicData.BP.Cn.Cn.dHT  ExtrapMethod=Linear
  C_N : Outport
  wires:
  [beta] -> Prelookup4/1  "beta"
  [alpha] -> Prelookup3/1  "alpha"
  Prelookup3/2 -> Interpolation Using Prelookup1/2
  [delta_e] -> Prelookup5/1  "dHT"
  Prelookup3/1 -> Interpolation Using Prelookup1/1
  Prelookup5/1 -> Interpolation Using Prelookup1/5
  Prelookup5/2 -> Interpolation Using Prelookup1/6
  Prelookup4/1 -> Interpolation Using Prelookup1/3
  Prelookup4/2 -> Interpolation Using Prelookup1/4
  Interpolation Using Prelookup1/1 -> C_N/1  "C_N"

== system project_simulink/Subsystem15/Subsystem1 ==
  Interpolation Using Prelookup3 : Interpolation_n-D  Table=f16_database.f16_AerodynamicData.data.Cn.Cnda20  InternalRulePriority=Speed
  Prelookup7 : PreLookup  BreakpointsData=f16_database.f16_AerodynamicData.BP.Cn.Cnda20.alpha  ExtrapMethod=Linear
  Prelookup8 : PreLookup  BreakpointsData=f16_database.f16_AerodynamicData.BP.Cn.Cnda20.beta  ExtrapMethod=Linear
  C_N_delta_a : Outport
  wires:
  [alpha] -> Prelookup7/1  "alpha"
  Prelookup8/1 -> Interpolation Using Prelookup3/3
  Prelookup7/1 -> Interpolation Using Prelookup3/1
  Interpolation Using Prelookup3/1 -> C_N_delta_a/1  "C_N_delta_a"
  [beta] -> Prelookup8/1  "beta"
  Prelookup8/2 -> Interpolation Using Prelookup3/4
  Prelookup7/2 -> Interpolation Using Prelookup3/2

== system project_simulink/Subsystem15/Subsystem11 ==
  Interpolation Using Prelookup9 : Interpolation_n-D  NumberOfTableDimensions=1  Table=f16_database.f16_AerodynamicData.data.Cn.deltaCnplef  InternalRulePriority=Speed
      settings: InputPortMap=u0,u1
  Prelookup16 : PreLookup  BreakpointsData=f16_database.f16_AerodynamicData.BP.Cn.deltaCnplef.alpha  ExtrapMethod=Linear
  C_N_p_LEF : Outport
  wires:
  Prelookup16/2 -> Interpolation Using Prelookup9/2
  Prelookup16/1 -> Interpolation Using Prelookup9/1
  Interpolation Using Prelookup9/1 -> C_N_p_LEF/1  "C_N_p_LEF"
  [alpha] -> Prelookup16/1  "alpha"

== system project_simulink/Subsystem15/Subsystem13 ==
  Interpolation Using Prelookup10 : Interpolation_n-D  NumberOfTableDimensions=1  Table=f16_database.f16_AerodynamicData.data.Cn.deltaCnBeta  InternalRulePriority=Speed
      settings: InputPortMap=u0,u1
  Prelookup17 : PreLookup  BreakpointsData=f16_database.f16_AerodynamicData.BP.Cn.deltaCnBeta.alpha  ExtrapMethod=Linear
  delta_C_N_beta : Outport
  wires:
  Prelookup17/2 -> Interpolation Using Prelookup10/2
  Prelookup17/1 -> Interpolation Using Prelookup10/1
  Interpolation Using Prelookup10/1 -> delta_C_N_beta/1  "delta_C_N_beta"
  [alpha] -> Prelookup17/1  "alpha"

== system project_simulink/Subsystem15/Subsystem14 ==
  Interpolation Using Prelookup11 : Interpolation_n-D  Table=f16_database.f16_AerodynamicData.data.Cn.Cnlef  InternalRulePriority=Speed
  Prelookup18 : PreLookup  BreakpointsData=f16_database.f16_AerodynamicData.BP.Cn.Cnlef.beta  ExtrapMethod=Linear
  Prelookup19 : PreLookup  BreakpointsData=f16_database.f16_AerodynamicData.BP.Cn.Cnlef.alpha  ExtrapMethod=Linear
  C_N_LEF : Outport
  wires:
  Prelookup19/2 -> Interpolation Using Prelookup11/2
  [beta] -> Prelookup18/1  "beta"
  [alpha] -> Prelookup19/1  "alpha"
  Prelookup18/1 -> Interpolation Using Prelookup11/3
  Prelookup18/2 -> Interpolation Using Prelookup11/4
  Interpolation Using Prelookup11/1 -> C_N_LEF/1  "C_N_LEF"
  Prelookup19/1 -> Interpolation Using Prelookup11/1

== system project_simulink/Subsystem15/Subsystem2 ==
  Constant6 : Constant  Value=0
  Interpolation Using Prelookup2 : Interpolation_n-D  NumberOfTableDimensions=3  Table=f16_database.f16_AerodynamicData.data.Cn.Cn  InternalRulePriority=Speed
      settings: InputPortMap=u0,u1,u2,u3,u4,u5
  Prelookup1 : PreLookup  BreakpointsData=f16_database.f16_AerodynamicData.BP.Cn.Cn.alpha  ExtrapMethod=Linear
  Prelookup2 : PreLookup  BreakpointsData=f16_database.f16_AerodynamicData.BP.Cn.Cn.beta  ExtrapMethod=Linear
  Prelookup6 : PreLookup  BreakpointsData=f16_database.f16_AerodynamicData.BP.Cn.Cn.dHT  ExtrapMethod=Linear
  C_N_HT0 : Outport
  wires:
  Prelookup1/2 -> Interpolation Using Prelookup2/2
  [alpha] -> Prelookup1/1  "alpha"
  Interpolation Using Prelookup2/1 -> C_N_HT0/1  "C_N_HT0"
  Constant6/1 -> Prelookup6/1  "dHT"
  Prelookup6/2 -> Interpolation Using Prelookup2/6
  [beta] -> Prelookup2/1  "beta"
  Prelookup1/1 -> Interpolation Using Prelookup2/1
  Prelookup2/1 -> Interpolation Using Prelookup2/3
  Prelookup2/2 -> Interpolation Using Prelookup2/4
  Prelookup6/1 -> Interpolation Using Prelookup2/5

== system project_simulink/Subsystem15/Subsystem3 ==
  Interpolation Using Prelookup4 : Interpolation_n-D  Table=f16_database.f16_AerodynamicData.data.Cn.Cnda20lef  InternalRulePriority=Speed
  Prelookup10 : PreLookup  BreakpointsData=f16_database.f16_AerodynamicData.BP.Cn.Cnda20lef.beta  ExtrapMethod=Linear
  Prelookup9 : PreLookup  BreakpointsData=f16_database.f16_AerodynamicData.BP.Cn.Cnda20lef.alpha  ExtrapMethod=Linear
  C_N_delta_a_LEF : Outport
  wires:
  Prelookup10/2 -> Interpolation Using Prelookup4/4
  Prelookup10/1 -> Interpolation Using Prelookup4/3
  Prelookup9/1 -> Interpolation Using Prelookup4/1
  [alpha] -> Prelookup9/1  "alpha"
  Prelookup9/2 -> Interpolation Using Prelookup4/2
  [beta] -> Prelookup10/1  "beta"
  Interpolation Using Prelookup4/1 -> C_N_delta_a_LEF/1  "C_N_delta_a_LEF"

== system project_simulink/Subsystem15/Subsystem4 ==
  Interpolation Using Prelookup5 : Interpolation_n-D  Table=f16_database.f16_AerodynamicData.data.Cn.Cndr30  InternalRulePriority=Speed
  Prelookup11 : PreLookup  BreakpointsData=f16_database.f16_AerodynamicData.BP.Cn.Cndr30.beta  ExtrapMethod=Linear
  Prelookup12 : PreLookup  BreakpointsData=f16_database.f16_AerodynamicData.BP.Cn.Cndr30.alpha  ExtrapMethod=Linear
  C_N_delta_r : Outport
  wires:
  [alpha] -> Prelookup12/1  "alpha"
  [beta] -> Prelookup11/1  "beta"
  Prelookup11/2 -> Interpolation Using Prelookup5/4
  Prelookup12/2 -> Interpolation Using Prelookup5/2
  Prelookup12/1 -> Interpolation Using Prelookup5/1
  Prelookup11/1 -> Interpolation Using Prelookup5/3
  Interpolation Using Prelookup5/1 -> C_N_delta_r/1  "C_N_delta_r"

== system project_simulink/Subsystem15/Subsystem5 ==
  Interpolation Using Prelookup7 : Interpolation_n-D  NumberOfTableDimensions=1  Table=f16_database.f16_AerodynamicData.data.Cn.Cnr  InternalRulePriority=Speed
      settings: InputPortMap=u0,u1
  Prelookup13 : PreLookup  BreakpointsData=f16_database.f16_AerodynamicData.BP.Cn.Cnr.alpha  ExtrapMethod=Linear
  C_N_r : Outport
  wires:
  Prelookup13/1 -> Interpolation Using Prelookup7/1
  Prelookup13/2 -> Interpolation Using Prelookup7/2
  [alpha] -> Prelookup13/1  "alpha"
  Interpolation Using Prelookup7/1 -> C_N_r/1  "C_N_r"

== system project_simulink/Subsystem15/Subsystem8 ==
  Interpolation Using Prelookup6 : Interpolation_n-D  NumberOfTableDimensions=1  Table=f16_database.f16_AerodynamicData.data.Cn.deltaCnrlef  InternalRulePriority=Speed
      settings: InputPortMap=u0,u1
  Prelookup14 : PreLookup  BreakpointsData=f16_database.f16_AerodynamicData.BP.Cn.deltaCnrlef.alpha  ExtrapMethod=Linear
  delta_C_N_r_LEF : Outport
  wires:
  Prelookup14/1 -> Interpolation Using Prelookup6/1
  [alpha] -> Prelookup14/1  "alpha"
  Prelookup14/2 -> Interpolation Using Prelookup6/2
  Interpolation Using Prelookup6/1 -> delta_C_N_r_LEF/1  "C_N_r_LEF"

== system project_simulink/Subsystem15/Subsystem9 ==
  Interpolation Using Prelookup8 : Interpolation_n-D  NumberOfTableDimensions=1  Table=f16_database.f16_AerodynamicData.data.Cn.Cnp  InternalRulePriority=Speed
      settings: InputPortMap=u0,u1
  Prelookup15 : PreLookup  BreakpointsData=f16_database.f16_AerodynamicData.BP.Cn.Cnp.alpha  ExtrapMethod=Linear
  C_N_p : Outport
  wires:
  [alpha] -> Prelookup15/1  "alpha"
  Prelookup15/1 -> Interpolation Using Prelookup8/1
  Interpolation Using Prelookup8/1 -> C_N_p/1  "C_N_p"
  Prelookup15/2 -> Interpolation Using Prelookup8/2

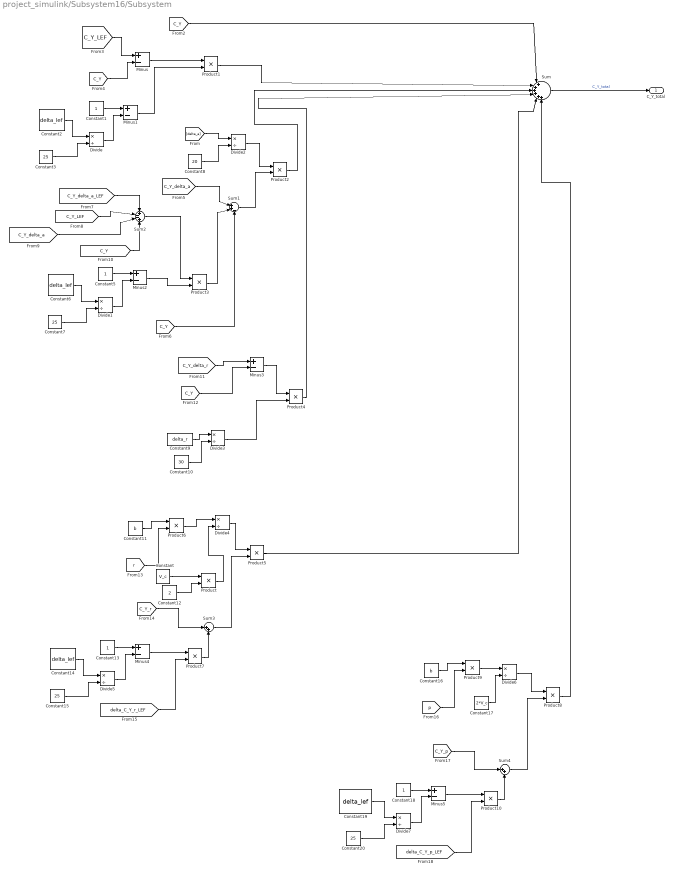
== system project_simulink/Subsystem16/Subsystem ==
  Constant : Constant  Value=V_c
  Constant{1,5,13,18} (4 alike) : Constant
  Constant10 : Constant  Value=30
  Constant11 : Constant  Value=b
  Constant12 : Constant  Value=2
  Constant{2,6,14,19} (4 alike) : Constant  Value=delta_lef
  Constant{3,7,15,20} (4 alike) : Constant  Value=25
  Constant16 : Constant  Value=b
  Constant17 : Constant  Value=2*V_c
  Constant8 : Constant  Value=20
  Constant9 : Constant  Value=delta_r
  Divide{,1..7} (8 alike) : Product  Inputs=*/
  Minus{,1..5} (6 alike) : Sum  Inputs=+-
  Product{,1..10} (11 alike) : Product
  Sum : Sum  Inputs=|++++++
  Sum1 : Sum  Inputs=|++-
  Sum2 : Sum  Inputs=+--+
  Sum3 : Sum  Inputs=|++
  Sum4 : Sum  Inputs=|++
  C_Y_total : Outport
  wires:
  Product10/1 -> Sum4/2
  Constant18/1 -> Minus5/1
  Constant14/1 -> Divide5/1
  Divide4/1 -> Product5/1
  [C_Y_LEF] -> Minus/1
  [C_Y] -> Sum1/3
  Constant11/1 -> Product6/1
  Constant8/1 -> Divide2/2
  [C_Y] -> Sum/1
  [C_Y_LEF] -> Sum2/2
  Minus1/1 -> Product1/2
  Constant9/1 -> Divide3/1
  Product1/1 -> Sum/2
  Constant15/1 -> Divide5/2
  Sum2/1 -> Product3/1
  Divide7/1 -> Minus5/2
  Divide2/1 -> Product2/1
  Minus/1 -> Product1/1
  [C_Y_delta_a] -> Sum1/1
  Constant7/1 -> Divide1/2
  Constant17/1 -> Divide6/2
  Minus4/1 -> Product7/1
  Product2/1 -> Sum/3
  Constant10/1 -> Divide3/2
  Product/1 -> Divide4/2
  Minus5/1 -> Product10/1
  Divide5/1 -> Minus4/2
  Constant13/1 -> Minus4/1
  [C_Y] -> Sum2/4
  [C_Y_delta_a] -> Sum2/3
  Product7/1 -> Sum3/2
  [r] -> Product6/2
  Divide6/1 -> Product8/1
  Constant16/1 -> Product9/1
  Constant19/1 -> Divide7/1
  Constant2/1 -> Divide/1
  Product9/1 -> Divide6/1
  Product3/1 -> Sum1/2
  Constant20/1 -> Divide7/2
  [C_Y] -> Minus3/2
  [C_Y_delta_r] -> Minus3/1
  [C_Y_delta_a_LEF] -> Sum2/1
  Product8/1 -> Sum/6
  [C_Y] -> Minus/2
  Sum1/1 -> Product2/2
  [delta_C_Y_p_LEF] -> Product10/2
  Product5/1 -> Sum/5
  Sum3/1 -> Product5/2
  [p] -> Product9/2
  [C_Y_r] -> Sum3/1
  Constant1/1 -> Minus1/1
  Product4/1 -> Sum/4
  [C_Y_p] -> Sum4/1
  Sum4/1 -> Product8/2
  Minus2/1 -> Product3/2
  Divide1/1 -> Minus2/2
  Constant5/1 -> Minus2/1
  Constant6/1 -> Divide1/1
  Minus3/1 -> Product4/1
  Product6/1 -> Divide4/1
  [delta_C_Y_r_LEF] -> Product7/2
  Constant3/1 -> Divide/2
  Divide/1 -> Minus1/2
  Divide3/1 -> Product4/2
  [delta_a] -> Divide2/1
  Sum/1 -> C_Y_total/1  "C_Y_total"
  Constant/1 -> Product/1
  Constant12/1 -> Product/2

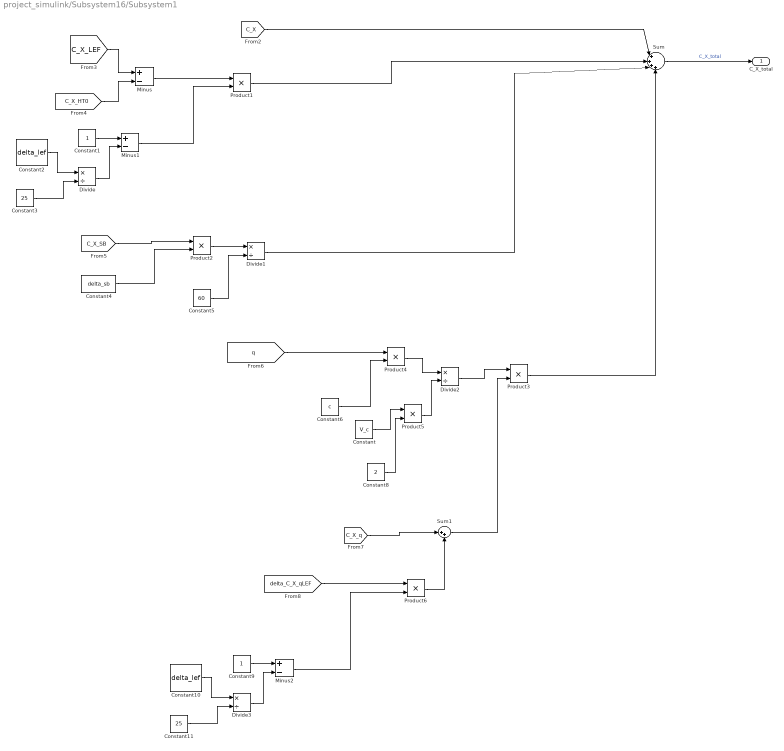
== system project_simulink/Subsystem16/Subsystem1 ==
  Constant : Constant  Value=V_c
  Constant1 : Constant
  Constant10 : Constant  Value=delta_lef
  Constant11 : Constant  Value=25
  Constant2 : Constant  Value=delta_lef
  Constant3 : Constant  Value=25
  Constant4 : Constant  Value=delta_sb
  Constant5 : Constant  Value=60
  Constant6 : Constant  Value=c
  Constant8 : Constant  Value=2
  Constant9 : Constant
  Divide{,1..3} (4 alike) : Product  Inputs=*/
  Minus : Sum  Inputs=+-
  Minus1 : Sum  Inputs=+-
  Minus2 : Sum  Inputs=+-
  Product{1..6} (6 alike) : Product
  Sum : Sum  Inputs=|++++
  Sum1 : Sum  Inputs=|++
  C_X_total : Outport
  wires:
  Product2/1 -> Divide1/1
  Product6/1 -> Sum1/2
  Constant6/1 -> Product4/2
  Product3/1 -> Sum/4
  [C_X_SB] -> Product2/1
  [C_X] -> Sum/1
  Constant9/1 -> Minus2/1
  Divide2/1 -> Product3/1
  Divide1/1 -> Sum/3
  [C_X_HT0] -> Minus/2
  Minus1/1 -> Product1/2
  Constant1/1 -> Minus1/1
  Constant5/1 -> Divide1/2
  Product5/1 -> Divide2/2
  Product4/1 -> Divide2/1
  Product1/1 -> Sum/2
  Minus/1 -> Product1/1
  Constant11/1 -> Divide3/2
  Constant4/1 -> Product2/2
  Constant8/1 -> Product5/2
  [C_X_LEF] -> Minus/1
  Divide3/1 -> Minus2/2
  Constant10/1 -> Divide3/1
  Minus2/1 -> Product6/2
  Constant/1 -> Product5/1
  [C_X_q] -> Sum1/1
  [delta_C_X_qLEF] -> Product6/1
  Sum1/1 -> Product3/2
  Sum/1 -> C_X_total/1  "C_X_total"
  Constant3/1 -> Divide/2
  Divide/1 -> Minus1/2
  Constant2/1 -> Divide/1
  [q] -> Product4/1

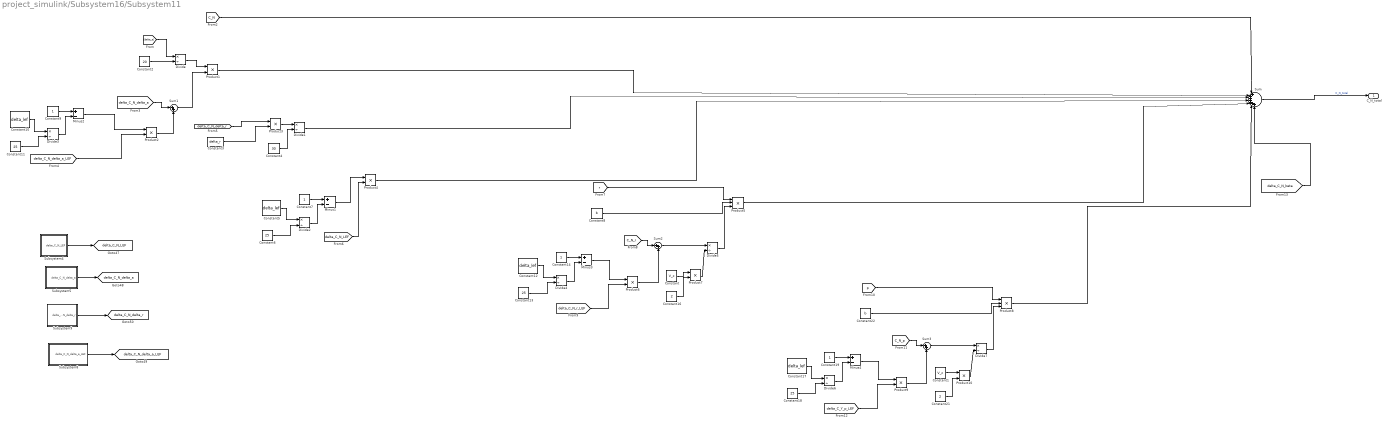
== system project_simulink/Subsystem16/Subsystem11 ==
  Constant : Constant  Value=V_c
  Constant1 : Constant  Value=V_c
  Constant{5,10,12,17} (4 alike) : Constant  Value=delta_lef
  Constant{6,11,13,18} (4 alike) : Constant  Value=25
  Constant{7,9,14,19} (4 alike) : Constant
  Constant16 : Constant  Value=2
  Constant2 : Constant  Value=20
  Constant21 : Constant  Value=2
  Constant22 : Constant  Value=b
  Constant3 : Constant  Value=delta_r
  Constant4 : Constant  Value=30
  Constant8 : Constant  Value=b
  Divide{,1..7} (8 alike) : Product  Inputs=*/
  Minus{1..4} (4 alike) : Sum  Inputs=+-
  Product{1..4,6..7,9..10} (8 alike) : Product
  Product5 : Product  Inputs=3
  Product8 : Product  Inputs=3
  Subsystem4 : Subsystem
  Subsystem5 : Subsystem
  Subsystem8 : Subsystem
  Subsystem9 : Subsystem
  Sum : Sum  Inputs=|+++++++
  Sum1 : Sum  Inputs=|++
  Sum2 : Sum  Inputs=|++
  Sum3 : Sum  Inputs=|++
  C_N_total : Outport
  tag scope: delta_C_N_LEF=global, delta_C_N_delta_a=global, delta_C_N_delta_a_LEF=global, delta_C_N_delta_r=global
  wires:
  Sum1/1 -> Product1/2
  [C_N_r] -> Sum2/1
  Product5/1 -> Sum/5
  Constant1/1 -> Product10/1
  [C_N_p] -> Sum3/1
  [C_N] -> Sum/1
  Product8/1 -> Sum/6
  Product3/1 -> Divide1/1
  Divide6/1 -> Minus4/2
  Divide1/1 -> Sum/3
  [delta_C_Y_p_LEF] -> Product9/2
  Constant2/1 -> Divide/2
  [delta_C_N_delta_a_LEF] -> Product2/2
  Constant21/1 -> Product10/2
  [r] -> Product5/1
  [delta_C_N_delta_a] -> Sum1/1
  Constant22/1 -> Product8/2
  Constant9/1 -> Minus2/1
  [delta_C_N_delta_r] -> Product3/1
  Product4/1 -> Sum/4
  Product10/1 -> Divide7/2
  Constant18/1 -> Divide6/2
  Divide/1 -> Product1/1
  Constant19/1 -> Minus4/1
  Constant7/1 -> Minus1/1
  [p] -> Product8/1
  Constant17/1 -> Divide6/1
  Divide4/1 -> Minus3/2
  Minus3/1 -> Product6/1
  [delta_C_N_r_LEF] -> Product6/2
  Constant16/1 -> Product7/2
  Minus2/1 -> Product2/1
  Divide3/1 -> Minus2/2
  Product9/1 -> Sum3/2
  Constant8/1 -> Product5/2
  Sum2/1 -> Divide5/1
  Divide7/1 -> Product8/3
  Sum/1 -> C_N_total/1  "C_N_total"
  Minus1/1 -> Product4/1
  Sum3/1 -> Divide7/1
  [delta_C_N_beta] -> Sum/7
  Constant11/1 -> Divide3/2
  Constant/1 -> Product7/1
  Product6/1 -> Sum2/2
  Constant10/1 -> Divide3/1
  Constant5/1 -> Divide2/1
  Divide2/1 -> Minus1/2
  Minus4/1 -> Product9/1
  Constant6/1 -> Divide2/2
  Constant14/1 -> Minus3/1
  [delta_C_N_LEF] -> Product4/2
  Divide5/1 -> Product5/3
  Constant12/1 -> Divide4/1
  Product1/1 -> Sum/2
  Constant13/1 -> Divide4/2
  [delta_a] -> Divide/1
  Product7/1 -> Divide5/2
  Constant3/1 -> Product3/2
  Constant4/1 -> Divide1/2
  Product2/1 -> Sum1/2
  Subsystem8/1(delta_C_N_delta_a_LEF) -> [delta_C_N_delta_a_LEF]
  Subsystem4/1(delta_C_N_LEF) -> [delta_C_N_LEF]
  Subsystem9/1(delta_C_N_delta_r) -> [delta_C_N_delta_r]
  Subsystem5/1(delta_C_N_delta_a) -> [delta_C_N_delta_a]

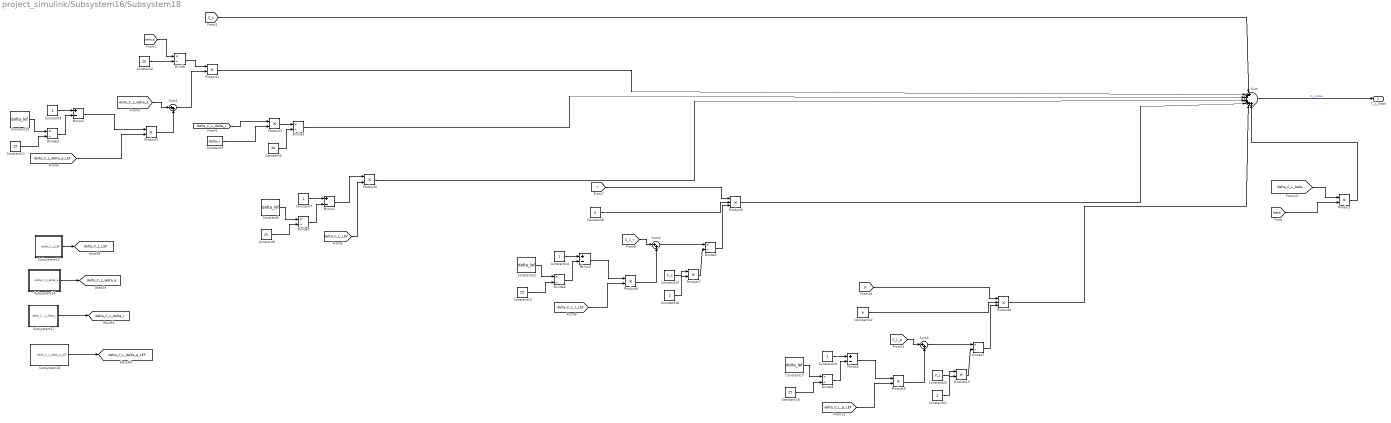
== system project_simulink/Subsystem16/Subsystem18 ==
  Constant{5,10,12,17} (4 alike) : Constant  Value=delta_lef
  Constant{6,11,13,18} (4 alike) : Constant  Value=25
  Constant{7,9,14,19} (4 alike) : Constant
  Constant15 : Constant  Value=V_c
  Constant16 : Constant  Value=2
  Constant2 : Constant  Value=20
  Constant20 : Constant  Value=V_c
  Constant21 : Constant  Value=2
  Constant22 : Constant  Value=b
  Constant3 : Constant  Value=delta_r
  Constant4 : Constant  Value=30
  Constant8 : Constant  Value=b
  Divide{,1..7} (8 alike) : Product  Inputs=*/
  Minus{1..4} (4 alike) : Sum  Inputs=+-
  Product{,1..4,6..7,9..10} (9 alike) : Product
  Product5 : Product  Inputs=3
  Product8 : Product  Inputs=3
  Subsystem13 : Subsystem
  Subsystem14 : Subsystem
  Subsystem16 : Subsystem
  Subsystem17 : Subsystem
  Sum : Sum  Inputs=|+++++++
  Sum1 : Sum  Inputs=|++
  Sum2 : Sum  Inputs=|++
  Sum3 : Sum  Inputs=|++
  C_L_total : Outport
  tag scope: delta_C_L_LEF=global, delta_C_L_delta_a=global, delta_C_L_delta_a_LEF=global, delta_C_L_delta_r=global
  wires:
  Product3/1 -> Divide1/1
  Constant8/1 -> Product5/2
  Constant5/1 -> Divide2/1
  Divide4/1 -> Minus3/2
  Product6/1 -> Sum2/2
  Constant14/1 -> Minus3/1
  [delta_C_L_delta_r] -> Product3/1
  [C_L] -> Sum/1
  Product4/1 -> Sum/4
  Product2/1 -> Sum1/2
  Minus4/1 -> Product9/1
  [delta_C_L_r_LEF] -> Product6/2
  Constant4/1 -> Divide1/2
  Constant3/1 -> Product3/2
  [delta_C_L_delta_a] -> Sum1/1
  [C_L_r] -> Sum2/1
  [C_L_p] -> Sum3/1
  Product5/1 -> Sum/5
  Sum1/1 -> Product1/2
  Constant10/1 -> Divide3/1
  Product7/1 -> Divide5/2
  Constant13/1 -> Divide4/2
  Constant20/1 -> Product10/1
  Product1/1 -> Sum/2
  Product10/1 -> Divide7/2
  [delta_C_L_delta_a_LEF] -> Product2/2
  [delta_C_L_p_LEF] -> Product9/2
  Divide2/1 -> Minus1/2
  Divide5/1 -> Product5/3
  Constant18/1 -> Divide6/2
  [delta_C_L_LEF] -> Product4/2
  Divide7/1 -> Product8/3
  Divide1/1 -> Sum/3
  Constant12/1 -> Divide4/1
  Product9/1 -> Sum3/2
  Minus2/1 -> Product2/1
  Sum2/1 -> Divide5/1
  [delta_a] -> Divide/1
  Constant6/1 -> Divide2/2
  [p] -> Product8/1
  Constant11/1 -> Divide3/2
  Sum3/1 -> Divide7/1
  Constant9/1 -> Minus2/1
  Sum/1 -> C_L_total/1  "C_L_total"
  Divide3/1 -> Minus2/2
  Minus3/1 -> Product6/1
  [r] -> Product5/1
  Product8/1 -> Sum/6
  Constant22/1 -> Product8/2
  Constant16/1 -> Product7/2
  Constant19/1 -> Minus4/1
  Constant17/1 -> Divide6/1
  Divide6/1 -> Minus4/2
  Divide/1 -> Product1/1
  Constant7/1 -> Minus1/1
  Minus1/1 -> Product4/1
  Constant15/1 -> Product7/1
  Constant2/1 -> Divide/2
  Constant21/1 -> Product10/2
  Subsystem16/1(delta_C_L_delta_a_LEF) -> [delta_C_L_delta_a_LEF]
  Subsystem14/1(delta_C_L_delta_a) -> [delta_C_L_delta_a]
  Subsystem13/1(delta_C_L_LEF) -> [delta_C_L_LEF]
  Subsystem17/1(delta_C_L_delta_r) -> [delta_C_L_delta_r]
  [delta_C_L_beta] -> Product/1
  [beta] -> Product/2
  Product/1 -> Sum/7
